simulink model "lab4_model"  (R2026a)
settings: Solver=VariableStepAuto
libraries: cstblocks_lti x2, simulink x1
settings Model: Creator=ms110  LastModifiedBy=ms110

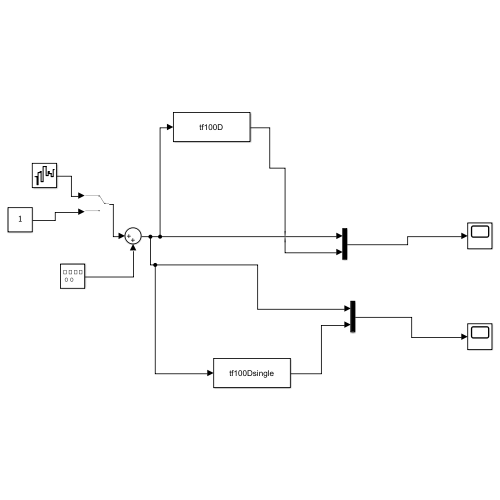
[thumbnail: Simulink's stored preview of the top-level diagram]
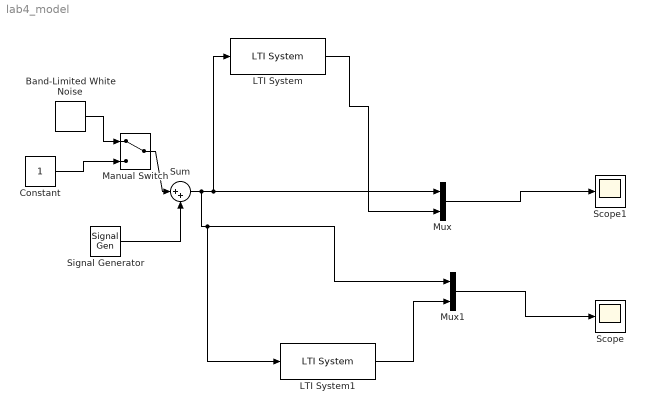
== system lab4_model ==
  Band-Limited White Noise : simulink/Sources/Band-Limited White Noise  Cov=[0.1]  Ts=0.1  seed=[23341]
  Constant : Constant
  LTI System : cstblocks_lti/LTI System  sys=tf100D  IC=[]  PadeOrder=0
      settings: LibrarySourceBlock=cstblocks/LTI System
  LTI System1 : cstblocks_lti/LTI System  sys=tf100Dsingle  IC=[]  PadeOrder=0
      settings: LibrarySourceBlock=cstblocks/LTI System
  Manual Switch : ManualSwitch
  Mux : Mux  Inputs=2
  Mux1 : Mux  Inputs=2
  Scope : Scope
  Scope1 : Scope
  Signal Generator : SignalGenerator  Units=rad/sec
  Sum : Sum  Inputs=|++
  wires:
  Constant/1 -> Manual Switch/2
  Band-Limited White Noise/1 -> Manual Switch/1
  Manual Switch/1 -> Sum/1
  Signal Generator/1 -> Sum/2
  Sum/1 -> LTI System1/1, Mux1/1, LTI System/1, Mux/1
  LTI System1/1 -> Mux1/2
  LTI System/1 -> Mux/2
  Mux/1 -> Scope1/1
  Mux1/1 -> Scope/1
